simulink model "ex_1"  (R2023b)
settings: Solver=FixedStepAuto  StartTime=0.0  StopTime=10.0  FixedStep=0.0001  RelTol=1e-3
settings Model: Creator=LucasDaiPráMartens  LastModifiedBy=LucasDaiPráMartens

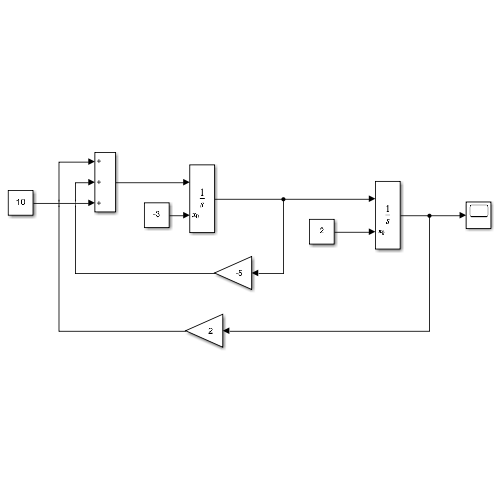
[thumbnail: Simulink's stored preview of the top-level diagram]
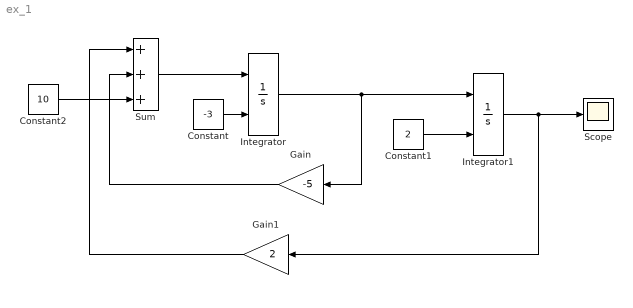
== system ex_1 ==
  Constant : Constant  Value=-3
  Constant1 : Constant  Value=2
  Constant2 : Constant  Value=10
  Gain : Gain  Gain=-5
  Gain1 : Gain  Gain=2
  Integrator : Integrator  InitialConditionSource=external
  Integrator1 : Integrator  InitialConditionSource=external
  Scope : Scope
  Sum : Sum  Inputs=+++
  wires:
  Integrator/1 -> Gain/1, Integrator1/1
  Constant/1 -> Integrator/2
  Gain1/1 -> Sum/1
  Sum/1 -> Integrator/1
  Constant1/1 -> Integrator1/2
  Gain/1 -> Sum/2
  Integrator1/1 -> Gain1/1, Scope/1
  Constant2/1 -> Sum/3
